simulink model "G_1"  (R2019a)
settings: Solver=VariableStepAuto  StartTime=0.0  StopTime=50  RelTol=1e-3
values from neighbouring files (symbols this model uses):
  A = sys_d.a    [ss2dt.m]    (also in vars.m = [[ 0.      0.      1.      0.    ])
  B = sys_d.b    [ss2dt.m]    (also in vars.m = [[0.        ])
  C = sys_d.c    [ss2dt.m]    (also in vars.m = [[1. 0. 0. 0.])
  K = [[ -2.00366979 199.78340569  -6.64587178  52.07504646]]    [vars.m]
  L = [[ 2.45    0.15  ] ... (first row only)    [vars.m]
libraries: commchan3 x1
settings Model: Creator=Artem  LastModifiedBy=Artem

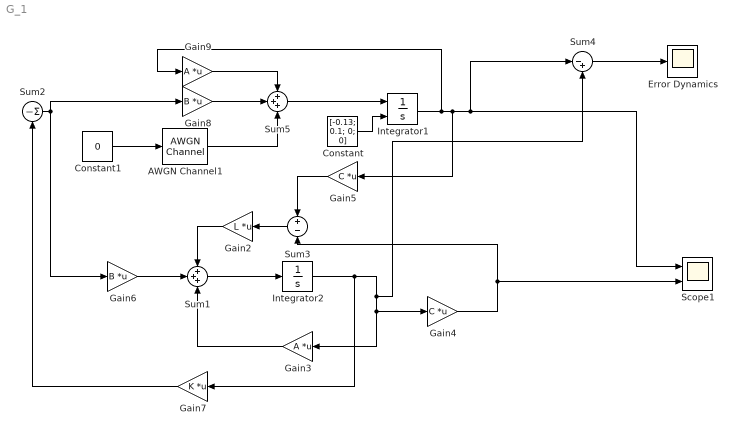
== system G_1 ==
  AWGN Channel1 : commchan3/AWGN Channel  InputProcessing=Columns as channels (frame based)  seed=2  noiseMode=Variance from mask  EbNodB=10  EsNodB=10  SNRdB=10  bitsPerSym=1  Ps=1  Tsym=1  variance=0.0001
      settings: SourceProductName=Communications Toolbox
  Constant : Constant  Value=[-0.13; 0.1; 0; 0]
  Constant1 : Constant  Value=0
  Error Dynamics : Scope
  Gain2 : Gain  Gain=L  Multiplication=Matrix(K*u)
  Gain3 : Gain  Gain=A  Multiplication=Matrix(K*u)
  Gain4 : Gain  Gain=C  Multiplication=Matrix(K*u)
  Gain5 : Gain  Gain=C  Multiplication=Matrix(K*u)
  Gain6 : Gain  Gain=B  Multiplication=Matrix(K*u)
  Gain7 : Gain  Gain=K  Multiplication=Matrix(K*u)
  Gain8 : Gain  Gain=B  Multiplication=Matrix(K*u)
  Gain9 : Gain  Gain=A  Multiplication=Matrix(K*u)
  Integrator1 : Integrator  InitialConditionSource=external
  Integrator2 : Integrator
  Scope1 : Scope  NumInputPorts=2
  Sum1 : Sum  Inputs=+++
  Sum2 : Sum  Inputs=||-
  Sum3 : Sum  Inputs=+-
  Sum4 : Sum  Inputs=|-+
  Sum5 : Sum  Inputs=+++
  wires:
  Gain7/1 -> Sum2/1
  Gain3/1 -> Sum1/3
  Gain5/1 -> Sum3/1
  Gain2/1 -> Sum1/1
  Sum3/1 -> Gain2/1
  Sum2/1 -> Gain6/1, Gain8/1
  Sum4/1 -> Error Dynamics/1
  Integrator2/1 -> Gain7/1, Sum4/2, Gain4/1, Gain3/1
  Gain4/1 -> Scope1/2, Sum3/2
  Sum1/1 -> Integrator2/1
  Integrator1/1 -> Gain9/1, Gain5/1, Scope1/1, Sum4/1
  Constant/1 -> Integrator1/2
  Sum5/1 -> Integrator1/1
  Gain6/1 -> Sum1/2
  Gain8/1 -> Sum5/2
  Gain9/1 -> Sum5/1
  Constant1/1 -> AWGN Channel1/1
  AWGN Channel1/1 -> Sum5/3
